simulink model "latlondist"  (R2022b)
settings: Solver=FixedStepAuto  StartTime=0.0  StopTime=10.0  FixedStep=1e-3  RelTol=1e-3
settings Model: Creator=asolland  LastModifiedBy=asolland
settings OptimizationCC: DefaultParameterBehavior=Inlined  EnhancedBackFolding=on  PassReuseOutputArgsAs=Individual arguments  OptimizeBlockOrder=speed  DifferentSizesBufferReuse=on  OptimizationCustomize=off  EfficientTunableParamExpr=on
settings DebuggingCC: ParameterTunabilityLossMsg=error
settings HardwareCC: TargetBitPerLong=64  TargetBitPerPointer=64  TargetBitPerSizeT=64  TargetBitPerPtrDiffT=64  TargetLongLongMode=on  TargetIntDivRoundTo=Zero  TargetEndianess=LittleEndian  TargetWordSize=64  TargetHWDeviceType=MATLAB Host  ProdEqTarget=off
settings SFSimCC: MATLABDynamicMemAlloc=off
settings RTWCC: Description=Embedded Coder (host-based shared library target)  SystemTargetFile=sim_pandas.tlc  TemplateMakefile=ert_default_tmf  GPUComputeCapability=5.0
settings CodeAppCC: ForceParamTrailComments=on  OperatorAnnotations=on  SimulinkDataObjDesc=on  SFDataObjDesc=on  InsertBlockDesc=on
settings STFCustomTargetCC: TargetLangStandard=C99 (ISO)  MultiwordLength=256  GenerateSampleERTMain=on  ParMdlRefBuildCompliant=on  CompOptLevelCompliant=on  CombineOutputUpdateFcns=on  ERTCustomFileBanners=on  CodeInterfacePackaging=Reusable function  SupportContinuousTime=off  SupportNonInlinedSFcns=off  RemoveResetFunc=on  MATLABClassNameForMDSCustomization=Simulink.SoftwareTarget.ERTCustomization  ModelStepFunctionPrototypeControlCompliant=on  UseToolchainInfoCompliant=on  SystemTargetFile=sim_pandas.tlc
settings ERTTargetCC: TargetLangStandard=C99 (ISO)  GenerateSampleERTMain=on  ConcurrentExecutionCompliant=off  CodeInterfacePackaging=Reusable function  CPPClassGenCompliant=off  InlinedParameterPlacement=NonHierarchical  RootIOFormat=Part of model data structure  ERTCustomFileTemplate=example_file_process.tlc

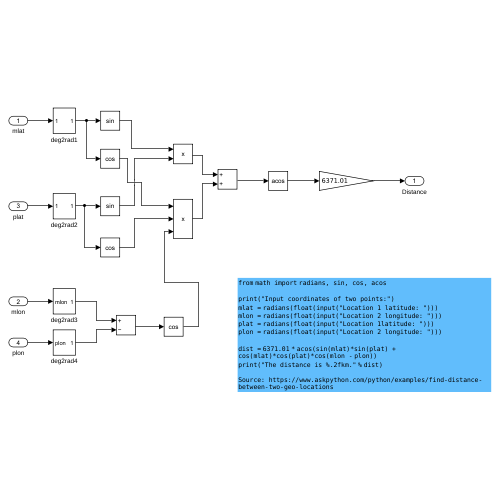
[thumbnail: Simulink's stored preview of the top-level diagram]
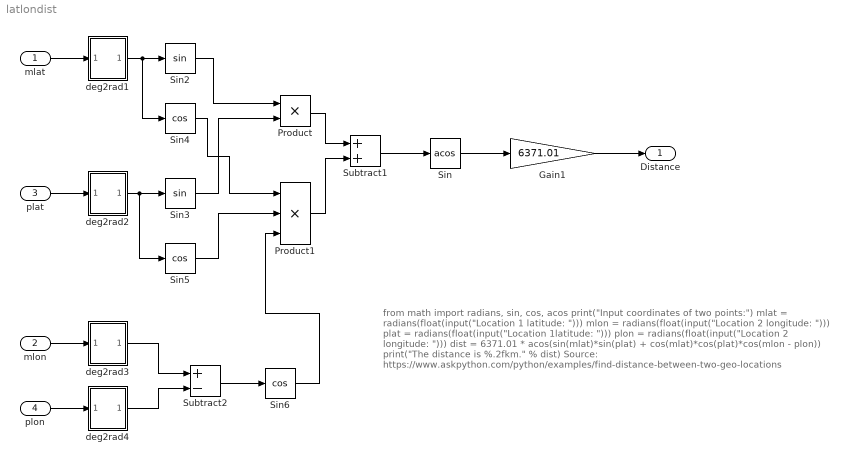
== system latlondist ==
  note: from math import radians, sin, cos, acos
      |
      | print("Input coordinates of two points:")
      | mlat = radians(float(input("Location 1 latitude: ")))
      | mlon = radians(float(input("Location 2 longitude: ")))
      | plat = radians(float(input("Location 1latitude: ")))
      | plon = radians(float(input("Location 2 longitude: ")))
      |
      | dist = 6371.01 * acos(sin(mlat)*sin(plat) + cos(mlat)*cos(plat)*cos(mlon - plon))
      | print("The distance is %.2fkm." % dist)
      |
      | Source: https://www.askpython.com/python/examples/find-distance-between-two-geo-locations
  mlat : Inport
  mlon : Inport  Port=2
  plat : Inport  Port=3
  plon : Inport  Port=4
  Gain1 : Gain  Gain=6371.01
  Product : Product
  Product1 : Product  Inputs=3
  Sin : Trigonometry  Operator=acos  OutputSignalType=real
  Sin2 : Trigonometry  OutputSignalType=real
  Sin3 : Trigonometry  OutputSignalType=real
  Sin4 : Trigonometry  Operator=cos  OutputSignalType=real
  Sin5 : Trigonometry  Operator=cos  OutputSignalType=real
  Sin6 : Trigonometry  Operator=cos  OutputSignalType=real
  Subtract1 : Sum
  Subtract2 : Sum  Inputs=+-
  deg2rad1 : Subsystem
  deg2rad2 : Subsystem
  deg2rad3 : Subsystem
  deg2rad4 : Subsystem
  Distance : Outport
  wires:
  mlat/1 -> deg2rad1/1(In1)
  plat/1 -> deg2rad2/1(In1)
  deg2rad1/1(Out1) -> Sin4/1, Sin2/1
  deg2rad2/1(Out1) -> Sin5/1, Sin3/1
  Sin2/1 -> Product/1
  Sin3/1 -> Product/2
  Sin4/1 -> Product1/1
  Sin5/1 -> Product1/2
  Product/1 -> Subtract1/1
  Product1/1 -> Subtract1/2
  mlon/1 -> deg2rad3/1(mlon)
  plon/1 -> deg2rad4/1(plon)
  deg2rad3/1(Out1) -> Subtract2/1
  deg2rad4/1(Out1) -> Subtract2/2
  Subtract2/1 -> Sin6/1
  Sin6/1 -> Product1/3
  Subtract1/1 -> Sin/1
  Sin/1 -> Gain1/1
  Gain1/1 -> Distance/1

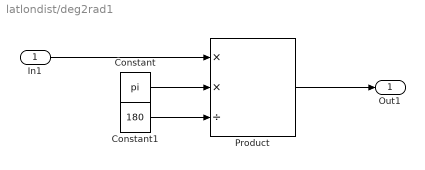
== system latlondist/deg2rad1 ==
  In1 : Inport
  Constant : Constant  Value=pi
  Constant1 : Constant  Value=180
  Product : Product  Inputs=**/
  Out1 : Outport
  wires:
  In1/1 -> Product/1
  Constant1/1 -> Product/3
  Constant/1 -> Product/2
  Product/1 -> Out1/1

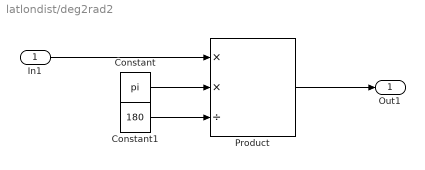
== system latlondist/deg2rad2 ==
  In1 : Inport
  Constant : Constant  Value=pi
  Constant1 : Constant  Value=180
  Product : Product  Inputs=**/
  Out1 : Outport
  wires:
  Product/1 -> Out1/1
  Constant/1 -> Product/2
  Constant1/1 -> Product/3
  In1/1 -> Product/1

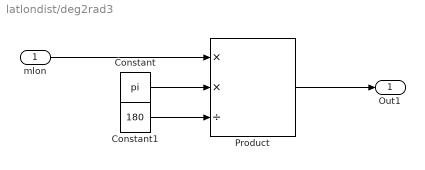
== system latlondist/deg2rad3 ==
  mlon : Inport
  Constant : Constant  Value=pi
  Constant1 : Constant  Value=180
  Product : Product  Inputs=**/
  Out1 : Outport
  wires:
  Product/1 -> Out1/1
  Constant/1 -> Product/2
  Constant1/1 -> Product/3
  mlon/1 -> Product/1

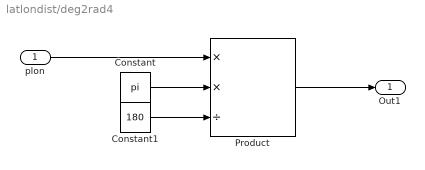
== system latlondist/deg2rad4 ==
  plon : Inport
  Constant : Constant  Value=pi
  Constant1 : Constant  Value=180
  Product : Product  Inputs=**/
  Out1 : Outport
  wires:
  plon/1 -> Product/1
  Constant1/1 -> Product/3
  Constant/1 -> Product/2
  Product/1 -> Out1/1
